simulink model "pneumo_hydraulic_Lyapunov"  (R2019b)
settings: Solver=VariableStepAuto  StartTime=0.0  StopTime=0.025  RelTol=1e-3
settings Model: Creator=User  LastModifiedBy=User

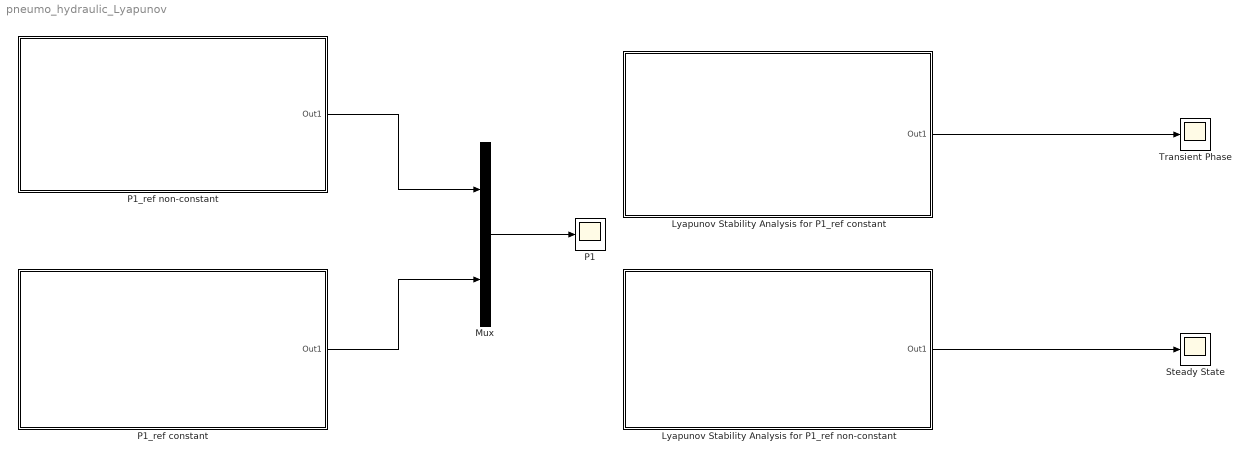
== system pneumo_hydraulic_Lyapunov ==
  Lyapunov Stability Analysis for P1_ref constant : Subsystem
  Lyapunov Stability Analysis for P1_ref non-constant : Subsystem
  Mux : Mux  Inputs=2
  P1 : Scope
  P1_ref constant : Subsystem
  P1_ref non-constant : Subsystem
  Steady State : Scope
  Transient Phase : Scope
  wires:
  P1_ref non-constant/1(Out1) -> Mux/1
  P1_ref constant/1(Out1) -> Mux/2
  Mux/1 -> P1/1
  Lyapunov Stability Analysis for P1_ref constant/1(Out1) -> Transient Phase/1
  Lyapunov Stability Analysis for P1_ref non-constant/1(Out1) -> Steady State/1

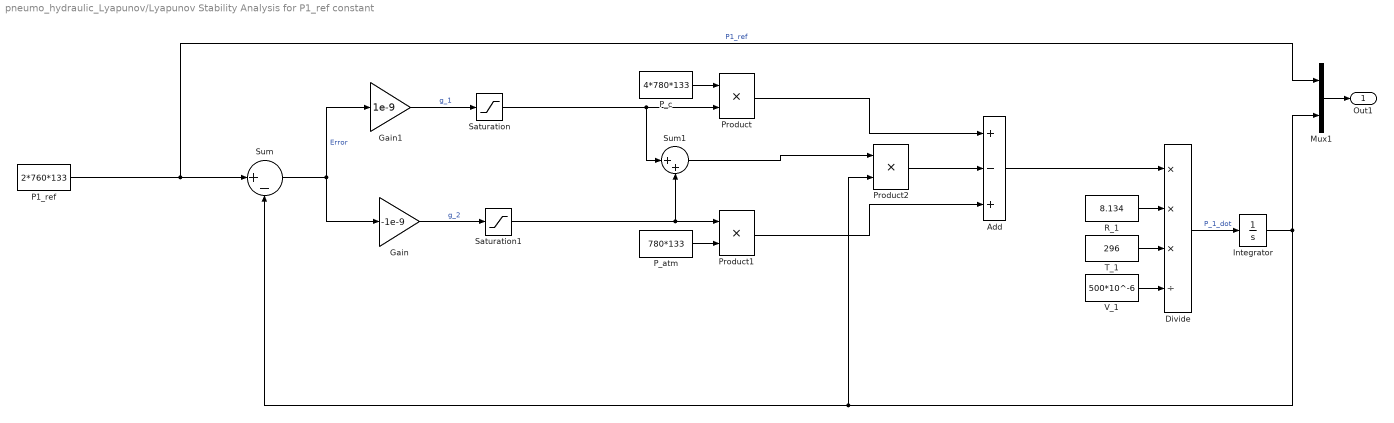
== system pneumo_hydraulic_Lyapunov/Lyapunov Stability Analysis for P1_ref constant ==
  Add : Sum  Inputs=+-+
  Divide : Product  Inputs=***/
  Gain : Gain  Gain=-1e-9
  Gain1 : Gain  Gain=1e-9
  Integrator : Integrator
  Mux1 : Mux  Inputs=2
  P1_ref : Constant  Value=2*760*133
  P_atm : Constant  Value=780*133
  P_c : Constant  Value=4*780*133
  Product : Product
  Product1 : Product
  Product2 : Product
  R_1 : Constant  Value=8.134
  Saturation : Saturate
  Saturation1 : Saturate
  Sum : Sum  Inputs=|+-
  Sum1 : Sum  Inputs=|++
  T_1 : Constant  Value=296
  V_1 : Constant  Value=500*10^-6
  Out1 : Outport
  wires:
  P_atm/1 -> Product1/2
  Product1/1 -> Add/3
  Integrator/1 -> Sum/2, Product2/2, Mux1/2
  Sum/1 -> Gain/1, Gain1/1  "Error"
  Gain1/1 -> Saturation/1  "g_1"
  Add/1 -> Divide/1
  V_1/1 -> Divide/4
  Product2/1 -> Add/2
  P_c/1 -> Product/1
  Divide/1 -> Integrator/1  "P_1_dot"
  Sum1/1 -> Product2/1
  T_1/1 -> Divide/3
  Product/1 -> Add/1
  Gain/1 -> Saturation1/1  "g_2"
  R_1/1 -> Divide/2
  Mux1/1 -> Out1/1
  Saturation/1 -> Sum1/1, Product/2
  Saturation1/1 -> Product1/1, Sum1/2
  P1_ref/1 -> Mux1/1, Sum/1  "P1_ref"

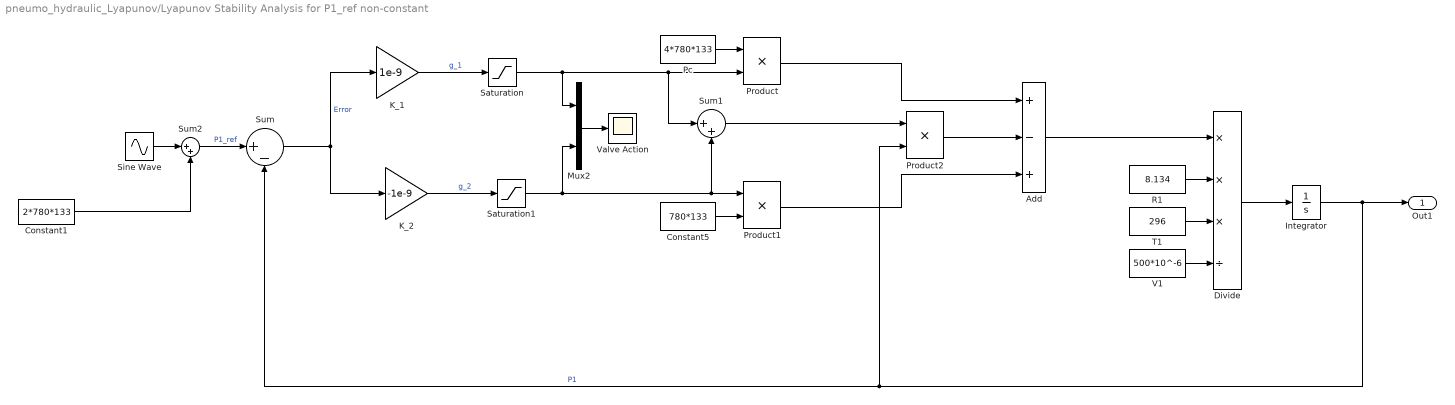
== system pneumo_hydraulic_Lyapunov/Lyapunov Stability Analysis for P1_ref non-constant ==
  Add : Sum  Inputs=+-+
  Constant1 : Constant  Value=2*780*133
  Constant5 : Constant  Value=780*133
  Divide : Product  Inputs=***/
  Integrator : Integrator
  K_1 : Gain  Gain=1e-9
  K_2 : Gain  Gain=-1e-9
  Mux2 : Mux  Inputs=2
  Pc : Constant  Value=4*780*133
  Product : Product
  Product1 : Product
  Product2 : Product
  R1 : Constant  Value=8.134
  Saturation : Saturate
  Saturation1 : Saturate
  Sine Wave : Sin  Amplitude=2*780*133  Frequency=1000  SampleTime=0
  Sum : Sum  Inputs=|+-
  Sum1 : Sum  Inputs=|++
  Sum2 : Sum  Inputs=|++
  T1 : Constant  Value=296
  V1 : Constant  Value=500*10^-6
  "Valve Action " : Scope
  Out1 : Outport
  wires:
  K_1/1 -> Saturation/1  "g_1"
  Mux2/1 -> "Valve Action "/1
  Integrator/1 -> Out1/1, Sum/2, Product2/2  "P1"
  Pc/1 -> Product/1
  Sum1/1 -> Product2/1
  V1/1 -> Divide/4
  Sum2/1 -> Sum/1  "P1_ref"
  Sine Wave/1 -> Sum2/1
  Saturation1/1 -> Mux2/2, Product1/1, Sum1/2
  Add/1 -> Divide/1
  Sum/1 -> K_2/1, K_1/1  "Error"
  Product2/1 -> Add/2
  Product1/1 -> Add/3
  K_2/1 -> Saturation1/1  "g_2"
  R1/1 -> Divide/2
  Saturation/1 -> Mux2/1, Sum1/1, Product/2
  Product/1 -> Add/1
  T1/1 -> Divide/3
  Constant5/1 -> Product1/2
  Divide/1 -> Integrator/1
  Constant1/1 -> Sum2/2

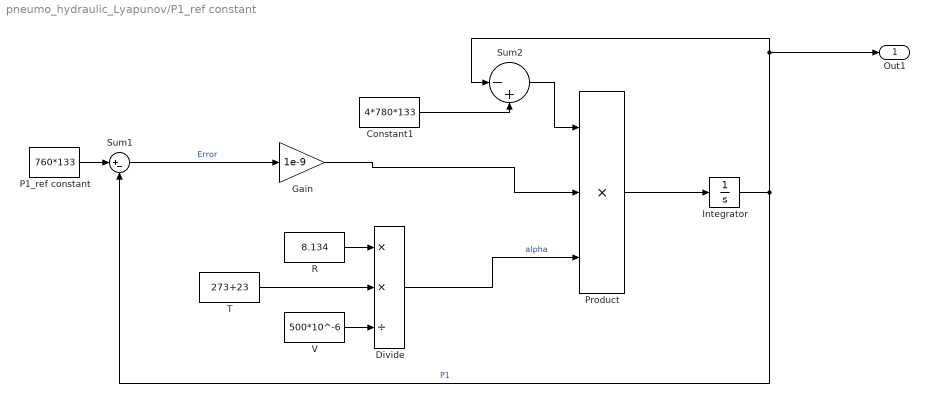
== system pneumo_hydraulic_Lyapunov/P1_ref constant ==
  Constant1 : Constant  Value=4*780*133
  Divide : Product  Inputs=**/
  Gain : Gain  Gain=1e-9
  Integrator : Integrator
  P1_ref constant : Constant  Value=760*133
  Product : Product  Inputs=3
  R : Constant  Value=8.134
  Sum1 : Sum  Inputs=|+-
  Sum2 : Sum  Inputs=|-+
  T : Constant  Value=273+23
  V : Constant  Value=500*10^-6
  Out1 : Outport
  wires:
  Product/1 -> Integrator/1
  Gain/1 -> Product/2
  Constant1/1 -> Sum2/2
  P1_ref constant/1 -> Sum1/1
  V/1 -> Divide/3
  Sum2/1 -> Product/1
  R/1 -> Divide/1
  Divide/1 -> Product/3  "alpha"
  Integrator/1 -> Sum1/2, Out1/1, Sum2/1  "P1"
  T/1 -> Divide/2
  Sum1/1 -> Gain/1  "Error"

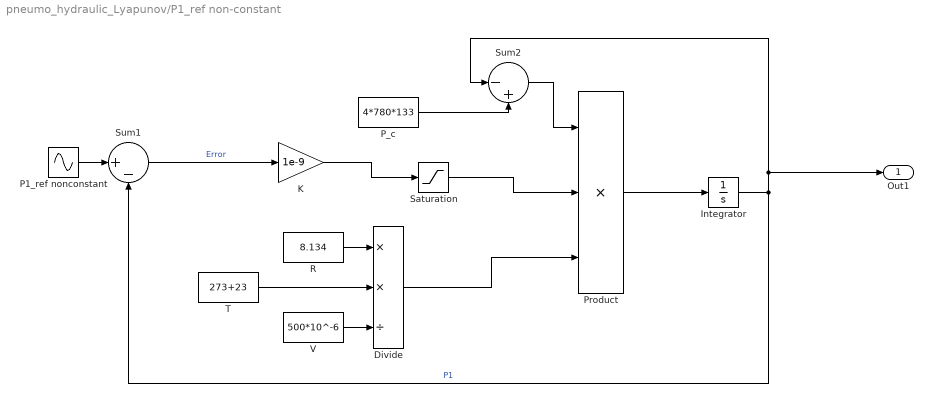
== system pneumo_hydraulic_Lyapunov/P1_ref non-constant ==
  Divide : Product  Inputs=**/
  Integrator : Integrator
  K : Gain  Gain=1e-9
  P1_ref nonconstant : Sin  Amplitude=760*133*1.15  Frequency=1000  SampleTime=0
  P_c : Constant  Value=4*780*133
  Product : Product  Inputs=3
  R : Constant  Value=8.134
  Saturation : Saturate
  Sum1 : Sum  Inputs=|+-
  Sum2 : Sum  Inputs=|-+
  T : Constant  Value=273+23
  V : Constant  Value=500*10^-6
  Out1 : Outport
  wires:
  P_c/1 -> Sum2/2
  Divide/1 -> Product/3
  R/1 -> Divide/1
  Integrator/1 -> Sum1/2, Sum2/1, Out1/1  "P1"
  Sum1/1 -> K/1  "Error"
  T/1 -> Divide/2
  V/1 -> Divide/3
  Product/1 -> Integrator/1
  Sum2/1 -> Product/1
  P1_ref nonconstant/1 -> Sum1/1
  K/1 -> Saturation/1
  Saturation/1 -> Product/2
